simulink model "teste_model"  (R2024b)
settings: Solver=FixedStepAuto  StartTime=0.0  StopTime=10.0  RelTol=1e-3
undefined symbols (not defined in the file): bool_on_off
settings Model: Creator=felipe  LastModifiedBy=felipe
settings OptimizationCC: PassReuseOutputArgsAs=Individual arguments  OptimizeBlockOrder=speed  DifferentSizesBufferReuse=on  EfficientTunableParamExpr=on
settings DebuggingCC: ParameterTunabilityLossMsg=error
settings HardwareCC: TargetBitPerLong=64  TargetBitPerPointer=64  TargetBitPerSizeT=64  TargetBitPerPtrDiffT=64  TargetLongLongMode=on  TargetIntDivRoundTo=Zero  TargetEndianess=LittleEndian  TargetWordSize=64  TargetHWDeviceType=MATLAB Host  ProdEqTarget=off
settings SFSimCC: MATLABDynamicMemAlloc=off
settings RTWCC: Description=Embedded Coder (host-based shared library target)  SystemTargetFile=ert_shrlib.tlc  TemplateMakefile=ert_default_tmf  RTWVerbose=off
settings RTWCC: CustomSourceCode=|
  | #define CONCAT(str1, str2, str3) CONCAT_(str1, str2, str3)
  | #define CONCAT_(str1, str2, str3) str1 ## str2 ## str3
  | #define GET_MMI_FUNC    CONCAT(MODEL     , _GetCAPImmi ,    )
  | #define RT_MODEL_STRUCT CONCAT(RT_MODEL_ , MODEL       , _T )
  | 
  | void* GET_MMI_FUNC(void* voidPtrToRealTimeStructure)
  | {
  |    rtwCAPI_ModelMappingInfo* mmiPtr = &(rtmGetDataMapInfo( ( RT_MODEL_STRUCT * )(voidPtrToRealTimeStructure) ).mmi);
  |    return (void*) mmiPtr;
  | }
settings CodeAppCC: GenerateComments=off  IgnoreCustomStorageClasses=off  OperatorAnnotations=on  SimulinkDataObjDesc=on  SFDataObjDesc=on  SimulinkBlockComments=off
settings STFCustomTargetCC: TargetLangStandard=C99 (ISO)  MultiwordLength=256  ParMdlRefBuildCompliant=on  CompOptLevelCompliant=on  IncludeMdlTerminateFcn=off  CombineOutputUpdateFcns=on  CombineSignalStateStructs=on  SuppressErrorStatus=on  ERTCustomFileBanners=on  SupportAbsoluteTime=off  CodeInterfacePackaging=Reusable function  SupportComplex=off  SupportContinuousTime=off  SupportNonInlinedSFcns=off  RemoveResetFunc=on  MATLABClassNameForMDSCustomization=Simulink.SoftwareTarget.ERTCustomization  ModelStepFunctionPrototypeControlCompliant=on  GenerateAllocFcn=on  UseToolchainInfoCompliant=on  SystemTargetFile=ert_shrlib.tlc
settings ERTTargetCC: TargetLangStandard=C99 (ISO)  ConcurrentExecutionCompliant=off  IncludeMdlTerminateFcn=off  CombineSignalStateStructs=on  SuppressErrorStatus=on  SupportAbsoluteTime=off  CodeInterfacePackaging=Reusable function  SupportComplex=off  CPPClassGenCompliant=off  GenerateAllocFcn=on  InlinedParameterPlacement=Hierarchical  RootIOFormat=Part of model data structure  RTWCAPIParams=on  RTWCAPIRootIO=on  ERTCustomFileTemplate=example_file_process.tlc

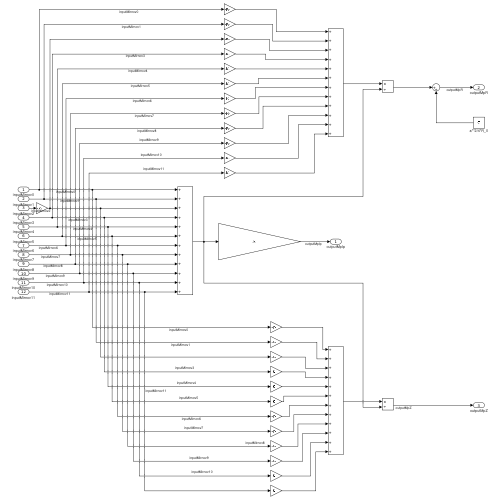
[thumbnail: Simulink's stored preview of the top-level diagram]
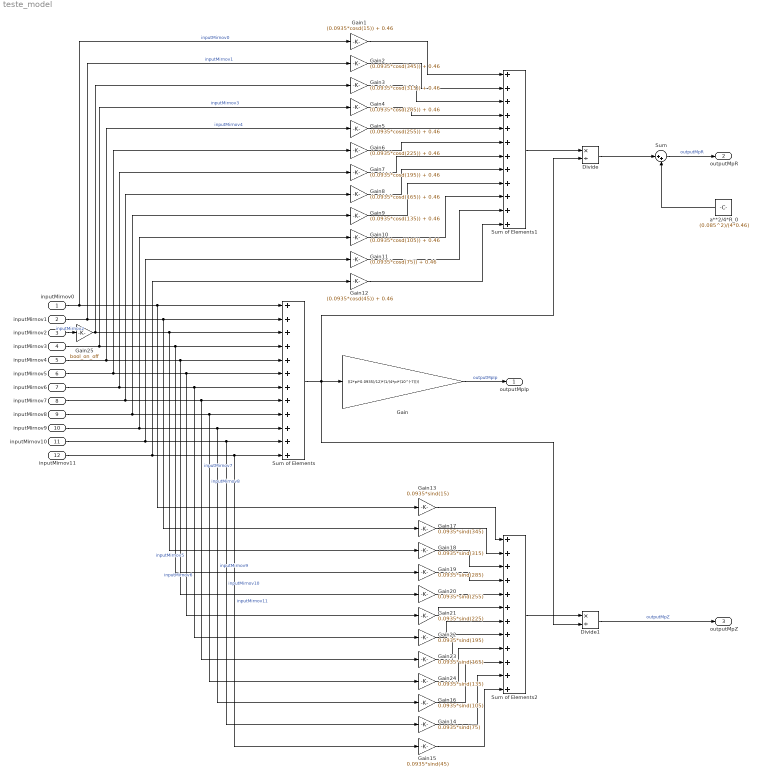
== system teste_model ==
  inputMirnov0 : Inport  OutDataTypeStr=double
  inputMirnov1 : Inport  Port=2  OutDataTypeStr=double
  inputMirnov2 : Inport  Port=3  OutDataTypeStr=double
  inputMirnov3 : Inport  Port=4  OutDataTypeStr=double
  inputMirnov4 : Inport  Port=5  OutDataTypeStr=double
  inputMirnov5 : Inport  Port=6  OutDataTypeStr=double
  inputMirnov6 : Inport  Port=7  OutDataTypeStr=double
  inputMirnov7 : Inport  Port=8  OutDataTypeStr=double
  inputMirnov8 : Inport  Port=9  OutDataTypeStr=double
  inputMirnov9 : Inport  Port=10  OutDataTypeStr=double
  inputMirnov10 : Inport  Port=11  OutDataTypeStr=double
  inputMirnov11 : Inport  Port=12  OutDataTypeStr=double
  Divide : Product  Inputs=*/
  Divide1 : Product  Inputs=*/
  Gain : Gain  Gain=((2*pi*0.0935)/12)*(1/(4*pi*(10^(-7))))
  Gain1 : Gain  Gain=(0.0935*cosd(15)) + 0.46
  Gain10 : Gain  Gain=(0.0935*cosd(105)) + 0.46
  Gain11 : Gain  Gain=(0.0935*cosd(75)) + 0.46
  Gain12 : Gain  Gain=(0.0935*cosd(45)) + 0.46
  Gain13 : Gain  Gain=0.0935*sind(15)
  Gain14 : Gain  Gain=0.0935*sind(75)
  Gain15 : Gain  Gain=0.0935*sind(45)
  Gain16 : Gain  Gain=0.0935*sind(105)
  Gain17 : Gain  Gain=0.0935*sind(345)
  Gain18 : Gain  Gain=0.0935*sind(315)
  Gain19 : Gain  Gain=0.0935*sind(285)
  Gain2 : Gain  Gain=(0.0935*cosd(345)) + 0.46
  Gain20 : Gain  Gain=0.0935*sind(255)
  Gain21 : Gain  Gain=0.0935*sind(225)
  Gain22 : Gain  Gain=0.0935*sind(195)
  Gain23 : Gain  Gain=0.0935*sind(165)
  Gain24 : Gain  Gain=0.0935*sind(135)
  Gain25 : Gain  Gain=bool_on_off
  Gain3 : Gain  Gain=(0.0935*cosd(315)) + 0.46
  Gain4 : Gain  Gain=(0.0935*cosd(285)) + 0.46
  Gain5 : Gain  Gain=(0.0935*cosd(255)) + 0.46
  Gain6 : Gain  Gain=(0.0935*cosd(225)) + 0.46
  Gain7 : Gain  Gain=(0.0935*cosd(195)) + 0.46
  Gain8 : Gain  Gain=(0.0935*cosd(165)) + 0.46
  Gain9 : Gain  Gain=(0.0935*cosd(135)) + 0.46
  Sum : Sum  Inputs=|++
  Sum of Elements : Sum  Inputs=++++++++++++
  Sum of Elements1 : Sum  Inputs=++++++++++++
  Sum of Elements2 : Sum  Inputs=++++++++++++
  a**2/4*R_0 : Constant  Value=(0.085^2)/(4*0.46)  OutDataTypeStr=double
  outputMpIp : Outport  OutDataTypeStr=double
  outputMpR : Outport  Port=2  OutDataTypeStr=double
  outputMpZ : Outport  Port=3  OutDataTypeStr=double
  wires:
  Sum of Elements2/1 -> Divide1/1
  Divide1/1 -> outputMpZ/1  "outputMpZ"
  inputMirnov6/1 -> Gain7/1, Gain22/1, Sum of Elements/7  "inputMirnov6"
  Gain19/1 -> Sum of Elements2/4
  Gain18/1 -> Sum of Elements2/3
  Gain12/1 -> Sum of Elements1/12
  Divide/1 -> Sum/1
  inputMirnov3/1 -> Gain4/1, Gain19/1, Sum of Elements/4  "inputMirnov3"
  Gain24/1 -> Sum of Elements2/9
  inputMirnov5/1 -> Gain6/1, Gain21/1, Sum of Elements/6  "inputMirnov5"
  inputMirnov4/1 -> Gain5/1, Gain20/1, Sum of Elements/5  "inputMirnov4"
  Gain11/1 -> Sum of Elements1/11
  Gain4/1 -> Sum of Elements1/4
  a**2/4*R_0/1 -> Sum/2
  inputMirnov8/1 -> Gain9/1, Gain24/1, Sum of Elements/9  "inputMirnov8"
  inputMirnov2/1 -> Gain25/1  "inputMirnov2"
  Gain23/1 -> Sum of Elements2/8
  Sum/1 -> outputMpR/1  "outputMpR"
  inputMirnov9/1 -> Gain10/1, Gain16/1, Sum of Elements/10  "inputMirnov9"
  Gain21/1 -> Sum of Elements2/6
  Gain5/1 -> Sum of Elements1/5
  inputMirnov1/1 -> Gain2/1, Gain17/1, Sum of Elements/2  "inputMirnov1"
  Gain3/1 -> Sum of Elements1/3
  Gain8/1 -> Sum of Elements1/8
  Gain20/1 -> Sum of Elements2/5
  Gain14/1 -> Sum of Elements2/11
  Gain17/1 -> Sum of Elements2/2
  Gain16/1 -> Sum of Elements2/10
  Gain22/1 -> Sum of Elements2/7
  Gain10/1 -> Sum of Elements1/10
  inputMirnov0/1 -> Gain1/1, Gain13/1, Sum of Elements/1  "inputMirnov0"
  Gain2/1 -> Sum of Elements1/2
  Gain15/1 -> Sum of Elements2/12
  inputMirnov10/1 -> Gain11/1, Gain14/1, Sum of Elements/11  "inputMirnov10"
  Gain6/1 -> Sum of Elements1/6
  Gain9/1 -> Sum of Elements1/9
  Sum of Elements1/1 -> Divide/1
  inputMirnov7/1 -> Gain8/1, Gain23/1, Sum of Elements/8  "inputMirnov7"
  Gain7/1 -> Sum of Elements1/7
  inputMirnov11/1 -> Gain12/1, Gain15/1, Sum of Elements/12  "inputMirnov11"
  Gain25/1 -> Gain3/1, Gain18/1, Sum of Elements/3
  Gain13/1 -> Sum of Elements2/1
  Gain1/1 -> Sum of Elements1/1
  Sum of Elements/1 -> Divide/2, Divide1/2, Gain/1
  Gain/1 -> outputMpIp/1  "outputMpIp"
